simulink subsystem "additive_biased_sensor"  (R2022a)
settings: Solver=VariableStepAuto  StartTime=0.0  StopTime=10.0  RelTol=1e-3
model mask{r=9 * 9.807 * 1e-3, rt=0, dt=0.01}
  mask prompts: r "RMS noise"; rt "Drift noise"; dt "Sample time [s]"
libraries: simulink x2
settings Model: Creator=yevge  LastModifiedBy=yevge

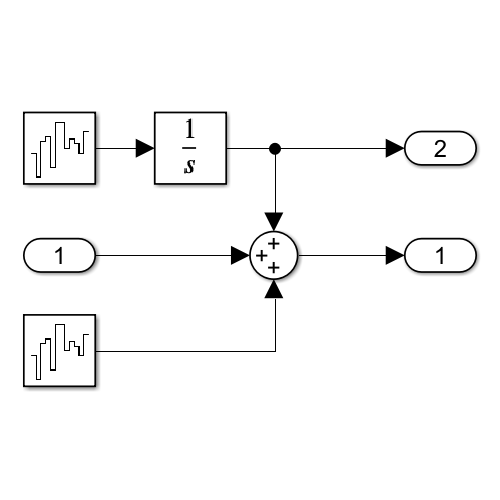
[thumbnail: Simulink's stored preview of the top-level diagram]
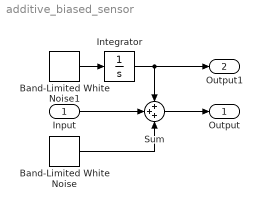
== system additive_biased_sensor ==
  Input : Inport
  Band-Limited White Noise : simulink/Sources/Band-Limited White Noise  Cov="r .^ 2  *dt"  Ts=dt  seed=randi(10000,1)
  Band-Limited White Noise1 : simulink/Sources/Band-Limited White Noise  Cov=rt .^2 * dt  Ts=dt  seed=randi(10000,1)
  Integrator : Integrator
  Sum : Sum  Inputs=+++
  Output : Outport
  Output1 : Outport  Port=2
  wires:
  Sum/1 -> Output/1
  Band-Limited White Noise1/1 -> Integrator/1
  Input/1 -> Sum/2
  Integrator/1 -> Output1/1, Sum/1
  Band-Limited White Noise/1 -> Sum/3
